simulink model "MPSK_in_AWGN"  (R2023a)
settings: Solver=VariableStepAuto  StartTime=0.0  StopTime=inf  RelTol=1e-3
values from neighbouring files (symbols this model uses):
  M = 2    [MPSK_control.m]
libraries: simulink x2, commsink2 x2, commdigbbndpm3 x2, commchan3 x1, commrandsrc3 x1
settings Model: SimulationMode=accelerator  Creator=arttu  LastModifiedBy=arttu
settings DataIOCC: ReturnWorkspaceOutputs=off

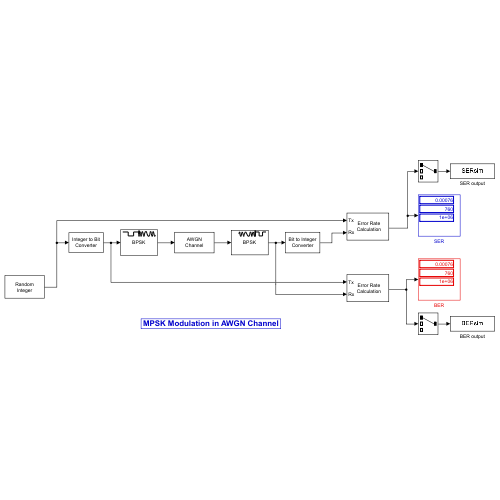
[thumbnail: Simulink's stored preview of the top-level diagram]
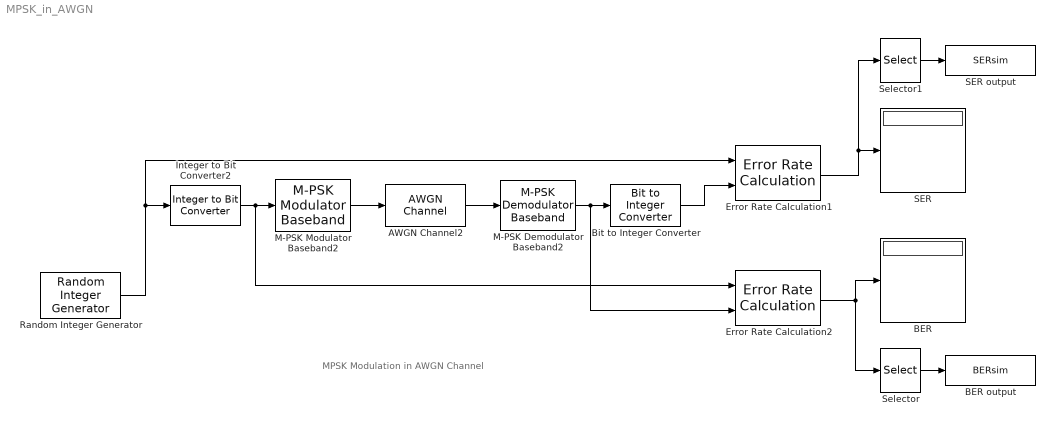
== system MPSK_in_AWGN ==
  note: MPSK Modulation in AWGN Channel
  AWGN Channel2 : commchan3/AWGN Channel  LegacyMode=on  NoiseMethod="Signal to noise ratio  (SNR)"  noiseMode="Signal to noise ratio  (Eb/No)"  EbNo=EbN0  EsNo=1 +10*log10(2)  SNR=0  BitsPerSymbol=log2(M)  SignalPower=1  SamplesPerSymbol=1  SymbolPeriod=1  VarianceSource=Parameter  Variance=1  RandomStream=Global stream  Seed=765432  SimulateUsing=Code generation
  BER : Display
  BER output : ToWorkspace  VariableName=BERsim  SaveFormat=Timeseries  SampleTime=-1
  Bit to Integer Converter : simulink/Logic and Bit Operations/Bit to Integer Converter  nbits=log2(M)  bitOrder=MSB first  signedOutputValues=Unsigned  outDtype=Same as input  outDtypeSigned=Inherit via internal rule
  Error Rate Calculation1 : commsink2/Error Rate Calculation  N=0  st_delay=0  cp_mode=Entire frame  subframe=[]  PMode=Port  WsName=ErrorVec  RsMode2=off  stop=on  numErr=1000  maxBits=1e6
  Error Rate Calculation2 : commsink2/Error Rate Calculation  N=0  st_delay=0  cp_mode=Entire frame  subframe=[]  PMode=Port  WsName=ErrorVec  RsMode2=off  stop=on  numErr=1000  maxBits=1e6
  Integer to Bit Converter2 : simulink/Logic and Bit Operations/Integer to Bit Converter  nbits=log2(M)  signedInputValues=Unsigned  bitOrder=MSB first  outDtype=Same as input
  M-PSK Demodulator Baseband2 : commdigbbndpm3/M-PSK Demodulator Baseband  M=M  OutType=Bit  DecType=Hard decision  VarSource=Dialog  Variance=1  Dec=Gray  Mapping=[0:7]  Ph=0  outDtype1=Inherit via internal rule  outDtype2=Inherit via internal rule  derotateFactorWordLen=16  derotateFactorDataTypeStr=Inherit: Same word length as input  derotateFactorLastDataTypeStr=Inherit: Same word length as input
  M-PSK Modulator Baseband2 : commdigbbndpm3/M-PSK Modulator Baseband  M=M  InType=Bit  Enc=Gray  Mapping=[0:7]  Ph=0  outDtype=double  outWordLen=16  outUDDataType=sfix(16)  outFracLenMode=Best precision  outFracLen=15  outDataTypeStr=double  outLastDataTypeStr=double
  Random Integer Generator : commrandsrc3/Random Integer Generator  SetSize=M  SeedSource=Parameter  Seed=234567  SampleTime=1  SamplesPerFrame=1  OutputDataType=double  SimulateUsing=Code generation
  SER : Display
  SER output : ToWorkspace  VariableName=SERsim  SaveFormat=Timeseries  SampleTime=-1
  Selector : Selector  InputPortWidth=3  IndexOptions=Index vector (dialog)  Indices=1  OutputSizes=1
  Selector1 : Selector  InputPortWidth=3  IndexOptions=Index vector (dialog)  Indices=1  OutputSizes=1
  wires:
  Error Rate Calculation2/1 -> Selector/1, BER/1
  Selector1/1 -> SER output/1
  Bit to Integer Converter/1 -> Error Rate Calculation1/2
  AWGN Channel2/1 -> M-PSK Demodulator Baseband2/1
  Random Integer Generator/1 -> Integer to Bit Converter2/1, Error Rate Calculation1/1
  Selector/1 -> BER output/1
  M-PSK Demodulator Baseband2/1 -> Error Rate Calculation2/2, Bit to Integer Converter/1
  Integer to Bit Converter2/1 -> M-PSK Modulator Baseband2/1, Error Rate Calculation2/1
  Error Rate Calculation1/1 -> SER/1, Selector1/1
  M-PSK Modulator Baseband2/1 -> AWGN Channel2/1
